simulink model "GolfSwing3D_SimscapePhysicalInterfaceSwitching"  (R2024b)
settings: Solver=VariableStepAuto  StartTime=0.0  StopTime=StopTime  MaxStep=0.001  RelTol=1e-3
model workspace: external: MAT-File 3DModelInputs.mat (data not in the file)
undefined symbols (not defined in the file): GripStrength, KillswitchFinalValue, KillswitchInitialValue, KillswitchStepTime, LeftLowerArmLength, PlaneTilt, RightLowerArmLength, UpperTorsoLength, X, Y, Z
libraries: nesl_utility x383, sm_lib x140, fl_lib x16, matrix_library x11, simulink x1
(part 9 of 14)

== system GolfSwing3D_SimscapePhysicalInterfaceSwitching/Right Scapula Joint/RScap Kinematically Driven ==
  Kinematically Driven RScap : sm_lib/Joints/Universal Joint  JointMode=Normal  CompositeWrenchDir=FollowerOnBase  CompositeWrenchFrame=BaseFrame  SenseConstraintForce=off  SenseConstraintTorque=off  SenseTotalForce=on  SenseTotalTorque=on  RxPositionTargetSpecify=off  RxPositionTargetPriority=Low  RxPositionTargetValue=RScapStartPositionX  RxPositionTargetValueUnits=deg  RxVelocityTargetSpecify=off  RxVelocityTargetPriority=Low  RxVelocityTargetValue=RScapStartVelocityX  RxVelocityTargetValueUnits=deg/s  RxEquilibriumPosition=0  RxEquilibriumPositionUnits=deg  RxSpringStiffness=0  RxSpringStiffnessUnits=N*m/deg  RxDampingCoefficient=0  RxDampingCoefficientUnits=N*m/(deg/s)  RxLowerLimitSpecify=off  RxLowerLimitBound=-30  RxLowerLimitBoundUnits=deg  RxLowerLimitStiffness=200  RxLowerLimitStiffnessUnits=N*m/deg  RxLowerLimitDamping=10  RxLowerLimitDampingUnits=N*m/(deg/s)  RxLowerLimitTransitionRegionWidth=0.1  RxLowerLimitTransitionRegionWidthUnits=deg  RxUpperLimitSpecify=off  RxUpperLimitBound=30  RxUpperLimitBoundUnits=deg  RxUpperLimitStiffness=200  RxUpperLimitStiffnessUnits=N*m/deg  RxUpperLimitDamping=10  RxUpperLimitDampingUnits=N*m/(deg/s)  RxUpperLimitTransitionRegionWidth=0.1  RxUpperLimitTransitionRegionWidthUnits=deg  RxTorqueActuationMode=ComputedTorque  RxMotionActuationMode=InputMotion  RxSensePosition=on  RxSenseVelocity=on  RxSenseAcceleration=off  RxSenseTorqueForce=on  RxSenseLowerLimitTorqueForce=off  RxSenseUpperLimitTorqueForce=off  RyPositionTargetSpecify=off  RyPositionTargetPriority=Low  RyPositionTargetValue=RScapStartPositionY  RyPositionTargetValueUnits=deg  RyVelocityTargetSpecify=off  RyVelocityTargetPriority=Low  RyVelocityTargetValue=RScapStartVelocityY  RyVelocityTargetValueUnits=deg/s  RyEquilibriumPosition=0  RyEquilibriumPositionUnits=deg  RySpringStiffness=0  RySpringStiffnessUnits=N*m/deg  RyDampingCoefficient=0  RyDampingCoefficientUnits=N*m/(deg/s)  RyLowerLimitSpecify=off  RyLowerLimitBound=-30  RyLowerLimitBoundUnits=deg  RyLowerLimitStiffness=200  RyLowerLimitStiffnessUnits=N*m/deg  RyLowerLimitDamping=10  RyLowerLimitDampingUnits=N*m/(deg/s)  RyLowerLimitTransitionRegionWidth=0.1  RyLowerLimitTransitionRegionWidthUnits=deg  RyUpperLimitSpecify=off  RyUpperLimitBound=30  RyUpperLimitBoundUnits=deg  RyUpperLimitStiffness=200  RyUpperLimitStiffnessUnits=N*m/deg  RyUpperLimitDamping=10  RyUpperLimitDampingUnits=N*m/(deg/s)  RyUpperLimitTransitionRegionWidth=0.1  RyUpperLimitTransitionRegionWidthUnits=deg  RyTorqueActuationMode=ComputedTorque  RyMotionActuationMode=InputMotion  RySensePosition=on  RySenseVelocity=on  RySenseAcceleration=off  RySenseTorqueForce=on  RySenseLowerLimitTorqueForce=off  RySenseUpperLimitTorqueForce=off
  RScapForceLocal : nesl_utility/PS-Simulink Converter  PhysicalDomain=network_engine_domain  SubClassName=ps_output  LeftPortType=input  RightPortType=output  PseudoPeriodic=off  Frequencies=[]  VectorFormat=1-D array  Unit=inherit  AffineConversion=off
  RScapPositionX : nesl_utility/PS-Simulink Converter  PhysicalDomain=network_engine_domain  SubClassName=ps_output  LeftPortType=input  RightPortType=output  PseudoPeriodic=off  Frequencies=[]  VectorFormat=1-D array  Unit=deg  AffineConversion=off
  RScapPositionY : nesl_utility/PS-Simulink Converter  PhysicalDomain=network_engine_domain  SubClassName=ps_output  LeftPortType=input  RightPortType=output  PseudoPeriodic=off  Frequencies=[]  VectorFormat=1-D array  Unit=deg  AffineConversion=off
  RScapTorqueLocal : nesl_utility/PS-Simulink Converter  PhysicalDomain=network_engine_domain  SubClassName=ps_output  LeftPortType=input  RightPortType=output  PseudoPeriodic=off  Frequencies=[]  VectorFormat=1-D array  Unit=inherit  AffineConversion=off
  RScapTorqueXInput : nesl_utility/PS-Simulink Converter  PhysicalDomain=network_engine_domain  SubClassName=ps_output  LeftPortType=input  RightPortType=output  PseudoPeriodic=off  Frequencies=[]  VectorFormat=1-D array  Unit=inherit  AffineConversion=off
  RScapTorqueYInput : nesl_utility/PS-Simulink Converter  PhysicalDomain=network_engine_domain  SubClassName=ps_output  LeftPortType=input  RightPortType=output  PseudoPeriodic=off  Frequencies=[]  VectorFormat=1-D array  Unit=inherit  AffineConversion=off
  RScapVelocityX : nesl_utility/PS-Simulink Converter  PhysicalDomain=network_engine_domain  SubClassName=ps_output  LeftPortType=input  RightPortType=output  PseudoPeriodic=off  Frequencies=[]  VectorFormat=1-D array  Unit=deg/s  AffineConversion=off
  RScapVelocityY : nesl_utility/PS-Simulink Converter  PhysicalDomain=network_engine_domain  SubClassName=ps_output  LeftPortType=input  RightPortType=output  PseudoPeriodic=off  Frequencies=[]  VectorFormat=1-D array  Unit=deg/s  AffineConversion=off
  Simulink-PS Converter14 : nesl_utility/Simulink-PS Converter  PhysicalDomain=network_engine_domain  SubClassName=ps_input  LeftPortType=input  RightPortType=output  PseudoPeriodic=off  Frequencies=[]  NoiseDistribution=none  NoiseParameters=[]  Unit=deg  AffineConversion=off  FilteringAndDerivatives=provide  SimscapeFilterOrder=1  InputFilterTimeConstant=0.001  UdotUserProvided=2
  Simulink-PS Converter15 : nesl_utility/Simulink-PS Converter  PhysicalDomain=network_engine_domain  SubClassName=ps_input  LeftPortType=input  RightPortType=output  PseudoPeriodic=off  Frequencies=[]  NoiseDistribution=none  NoiseParameters=[]  Unit=deg  AffineConversion=off  FilteringAndDerivatives=provide  SimscapeFilterOrder=1  InputFilterTimeConstant=0.001  UdotUserProvided=2
  Conn1 : PMIOPort  Side=Right
  Conn2 : PMIOPort  Port=2  Side=Left
  tag scope: RScapPositionX=global, RScapPositionY=global, RScapVelocityX=global, RScapVelocityY=global
  wires:
  [FcnOutRScapAccelerationY] -> Simulink-PS Converter15/3
  RScapPositionX/1 -> [RScapPositionX]  "RScapPositionX"
  RScapVelocityX/1 -> [RScapVelocityX]  "RScapVelocityX"
  [FcnOutRScapAccelerationX] -> Simulink-PS Converter14/3
  [FcnOutRScapPositionY] -> Simulink-PS Converter15/1
  RScapVelocityY/1 -> [RScapVelocityY]  "RScapVelocityY"
  RScapPositionY/1 -> [RScapPositionY]  "RScapPositionY"
  [FcnOutRScapPositionX] -> Simulink-PS Converter14/1
  [FcnOutRScapVelocityY] -> Simulink-PS Converter15/2
  [FcnOutRScapVelocityX] -> Simulink-PS Converter14/2
  RScapForceLocal/1 -> ?  "RScapForceLocal"
  RScapTorqueLocal/1 -> ?  "RScapTorqueLocal"
  RScapTorqueXInput/1 -> ?  "RScapTorqueXInput"
  RScapTorqueYInput/1 -> ?  "RScapTorqueYInput"
  connections:
  RScapVelocityX/LConn1 -- Kinematically Driven RScap/RConn3
  RScapPositionX/LConn1 -- Kinematically Driven RScap/RConn2
  Kinematically Driven RScap/RConn1 -- Conn1/RConn1
  RScapForceLocal/LConn1 -- Kinematically Driven RScap/RConn8
  Simulink-PS Converter15/RConn1 -- Kinematically Driven RScap/LConn3
  RScapVelocityY/LConn1 -- Kinematically Driven RScap/RConn6
  Simulink-PS Converter14/RConn1 -- Kinematically Driven RScap/LConn2
  RScapTorqueLocal/LConn1 -- Kinematically Driven RScap/RConn9
  RScapPositionY/LConn1 -- Kinematically Driven RScap/RConn5
  Kinematically Driven RScap/LConn1 -- Conn2/RConn1
  RScapTorqueYInput/LConn1 -- Kinematically Driven RScap/RConn7
  RScapTorqueXInput/LConn1 -- Kinematically Driven RScap/RConn4

== system GolfSwing3D_SimscapePhysicalInterfaceSwitching/Right Scapula Joint/RScap Kinetically Driven ==
  Kinetically Driven RScap : sm_lib/Joints/Universal Joint  JointMode=Normal  CompositeWrenchDir=FollowerOnBase  CompositeWrenchFrame=BaseFrame  SenseConstraintForce=off  SenseConstraintTorque=off  SenseTotalForce=on  SenseTotalTorque=on  RxPositionTargetSpecify=on  RxPositionTargetPriority=Low  RxPositionTargetValue=RScapStartPositionX  RxPositionTargetValueUnits=deg  RxVelocityTargetSpecify=off  RxVelocityTargetPriority=Low  RxVelocityTargetValue=RScapStartVelocityX  RxVelocityTargetValueUnits=deg/s  RxEquilibriumPosition=0  RxEquilibriumPositionUnits=deg  RxSpringStiffness=0  RxSpringStiffnessUnits=N*m/deg  RxDampingCoefficient=0  RxDampingCoefficientUnits=N*m/(deg/s)  RxLowerLimitSpecify=off  RxLowerLimitBound=-30  RxLowerLimitBoundUnits=deg  RxLowerLimitStiffness=200  RxLowerLimitStiffnessUnits=N*m/deg  RxLowerLimitDamping=10  RxLowerLimitDampingUnits=N*m/(deg/s)  RxLowerLimitTransitionRegionWidth=0.1  RxLowerLimitTransitionRegionWidthUnits=deg  RxUpperLimitSpecify=off  RxUpperLimitBound=30  RxUpperLimitBoundUnits=deg  RxUpperLimitStiffness=200  RxUpperLimitStiffnessUnits=N*m/deg  RxUpperLimitDamping=10  RxUpperLimitDampingUnits=N*m/(deg/s)  RxUpperLimitTransitionRegionWidth=0.1  RxUpperLimitTransitionRegionWidthUnits=deg  RxTorqueActuationMode=InputTorque  RxMotionActuationMode=ComputedMotion  RxSensePosition=on  RxSenseVelocity=on  RxSenseAcceleration=off  RxSenseTorqueForce=on  RxSenseLowerLimitTorqueForce=off  RxSenseUpperLimitTorqueForce=off  RyPositionTargetSpecify=on  RyPositionTargetPriority=Low  RyPositionTargetValue=RScapStartPositionY  RyPositionTargetValueUnits=deg  RyVelocityTargetSpecify=off  RyVelocityTargetPriority=Low  RyVelocityTargetValue=RScapStartVelocityY  RyVelocityTargetValueUnits=deg/s  RyEquilibriumPosition=0  RyEquilibriumPositionUnits=deg  RySpringStiffness=0  RySpringStiffnessUnits=N*m/deg  RyDampingCoefficient=0  RyDampingCoefficientUnits=N*m/(deg/s)  RyLowerLimitSpecify=off  RyLowerLimitBound=-30  RyLowerLimitBoundUnits=deg  RyLowerLimitStiffness=200  RyLowerLimitStiffnessUnits=N*m/deg  RyLowerLimitDamping=10  RyLowerLimitDampingUnits=N*m/(deg/s)  RyLowerLimitTransitionRegionWidth=0.1  RyLowerLimitTransitionRegionWidthUnits=deg  RyUpperLimitSpecify=off  RyUpperLimitBound=30  RyUpperLimitBoundUnits=deg  RyUpperLimitStiffness=200  RyUpperLimitStiffnessUnits=N*m/deg  RyUpperLimitDamping=10  RyUpperLimitDampingUnits=N*m/(deg/s)  RyUpperLimitTransitionRegionWidth=0.1  RyUpperLimitTransitionRegionWidthUnits=deg  RyTorqueActuationMode=InputTorque  RyMotionActuationMode=ComputedMotion  RySensePosition=on  RySenseVelocity=on  RySenseAcceleration=off  RySenseTorqueForce=on  RySenseLowerLimitTorqueForce=off  RySenseUpperLimitTorqueForce=off
  RScapForceLocal : nesl_utility/PS-Simulink Converter  PhysicalDomain=network_engine_domain  SubClassName=ps_output  LeftPortType=input  RightPortType=output  PseudoPeriodic=off  Frequencies=[]  VectorFormat=1-D array  Unit=inherit  AffineConversion=off
  RScapPositionX : nesl_utility/PS-Simulink Converter  PhysicalDomain=network_engine_domain  SubClassName=ps_output  LeftPortType=input  RightPortType=output  PseudoPeriodic=off  Frequencies=[]  VectorFormat=1-D array  Unit=deg  AffineConversion=off
  RScapPositionY : nesl_utility/PS-Simulink Converter  PhysicalDomain=network_engine_domain  SubClassName=ps_output  LeftPortType=input  RightPortType=output  PseudoPeriodic=off  Frequencies=[]  VectorFormat=1-D array  Unit=deg  AffineConversion=off
  RScapTorque : nesl_utility/PS-Simulink Converter  PhysicalDomain=network_engine_domain  SubClassName=ps_output  LeftPortType=input  RightPortType=output  PseudoPeriodic=off  Frequencies=[]  VectorFormat=1-D array  Unit=inherit  AffineConversion=off
  RScapTorqueXInput : nesl_utility/PS-Simulink Converter  PhysicalDomain=network_engine_domain  SubClassName=ps_output  LeftPortType=input  RightPortType=output  PseudoPeriodic=off  Frequencies=[]  VectorFormat=1-D array  Unit=inherit  AffineConversion=off
  RScapTorqueYInput : nesl_utility/PS-Simulink Converter  PhysicalDomain=network_engine_domain  SubClassName=ps_output  LeftPortType=input  RightPortType=output  PseudoPeriodic=off  Frequencies=[]  VectorFormat=1-D array  Unit=inherit  AffineConversion=off
  RScapVelocityX : nesl_utility/PS-Simulink Converter  PhysicalDomain=network_engine_domain  SubClassName=ps_output  LeftPortType=input  RightPortType=output  PseudoPeriodic=off  Frequencies=[]  VectorFormat=1-D array  Unit=deg/s  AffineConversion=off
  RScapVelocityY : nesl_utility/PS-Simulink Converter  PhysicalDomain=network_engine_domain  SubClassName=ps_output  LeftPortType=input  RightPortType=output  PseudoPeriodic=off  Frequencies=[]  VectorFormat=1-D array  Unit=deg/s  AffineConversion=off
  RightScapTorqueX : nesl_utility/Simulink-PS Converter  PhysicalDomain=network_engine_domain  SubClassName=ps_input  LeftPortType=input  RightPortType=output  PseudoPeriodic=off  Frequencies=[]  NoiseDistribution=none  NoiseParameters=[]  Unit=N*m  AffineConversion=off  FilteringAndDerivatives=provide  SimscapeFilterOrder=1  InputFilterTimeConstant=0.001  UdotUserProvided=0
  RightScapTorqueY : nesl_utility/Simulink-PS Converter  PhysicalDomain=network_engine_domain  SubClassName=ps_input  LeftPortType=input  RightPortType=output  PseudoPeriodic=off  Frequencies=[]  NoiseDistribution=none  NoiseParameters=[]  Unit=N*m  AffineConversion=off  FilteringAndDerivatives=provide  SimscapeFilterOrder=1  InputFilterTimeConstant=0.001  UdotUserProvided=0
  Conn1 : PMIOPort  Side=Left
  Conn2 : PMIOPort  Port=2  Side=Right
  tag scope: RScapPositionX=global, RScapPositionY=global, RScapVelocityX=global, RScapVelocityY=global
  wires:
  RScapPositionY/1 -> [RScapPositionY]  "RScapPositionY"
  [FcnOutRScapTorqueY] -> RightScapTorqueY/1
  [FcnOutRScapTorqueX] -> RightScapTorqueX/1
  RScapVelocityY/1 -> [RScapVelocityY]  "RScapVelocityY"
  RScapVelocityX/1 -> [RScapVelocityX]  "RScapVelocityX"
  RScapPositionX/1 -> [RScapPositionX]  "RScapPositionX"
  RScapTorque/1 -> ?  "RScapTorqueLocal"
  RScapForceLocal/1 -> ?  "RScapForceLocal"
  RScapTorqueXInput/1 -> ?  "RScapTorqueXInput"
  RScapTorqueYInput/1 -> ?  "RScapTorqueYInput"
  connections:
  Kinetically Driven RScap/LConn2 -- RightScapTorqueX/RConn1
  Kinetically Driven RScap/RConn3 -- RScapVelocityX/LConn1
  Kinetically Driven RScap/RConn6 -- RScapVelocityY/LConn1
  RScapForceLocal/LConn1 -- Kinetically Driven RScap/RConn8
  RScapTorque/LConn1 -- Kinetically Driven RScap/RConn9
  Kinetically Driven RScap/RConn2 -- RScapPositionX/LConn1
  RightScapTorqueY/RConn1 -- Kinetically Driven RScap/LConn3
  Kinetically Driven RScap/RConn5 -- RScapPositionY/LConn1
  Kinetically Driven RScap/LConn1 -- Conn1/RConn1
  Conn2/RConn1 -- Kinetically Driven RScap/RConn1
  RScapTorqueXInput/LConn1 -- Kinetically Driven RScap/RConn4
  RScapTorqueYInput/LConn1 -- Kinetically Driven RScap/RConn7

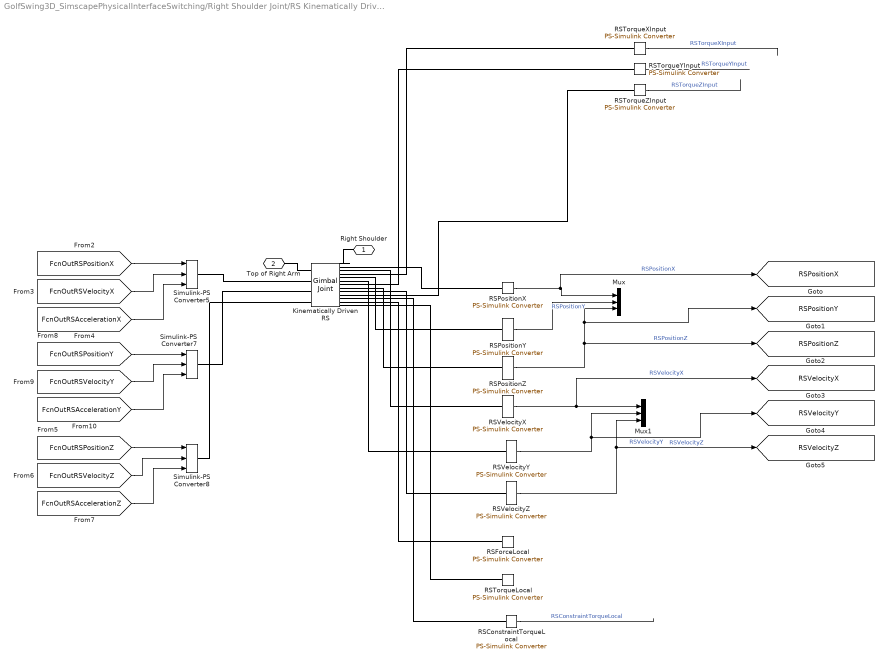
== system GolfSwing3D_SimscapePhysicalInterfaceSwitching/Right Shoulder Joint/RS Kinematically Driven ==
  Kinematically Driven RS : sm_lib/Joints/Gimbal Joint  JointMode=Normal  CompositeWrenchDir=BaseOnFollower  CompositeWrenchFrame=FollowerFrame  SenseConstraintForce=off  SenseConstraintTorque=on  SenseTotalForce=on  SenseTotalTorque=on  RxPositionTargetSpecify=off  RxPositionTargetPriority=Low  RxPositionTargetValue=RSStartPositionX  RxPositionTargetValueUnits=deg  RxVelocityTargetSpecify=off  RxVelocityTargetPriority=Low  RxVelocityTargetValue=RSStartVelocityX  RxVelocityTargetValueUnits=deg/s  RxEquilibriumPosition=120  RxEquilibriumPositionUnits=deg  RxSpringStiffness=0  RxSpringStiffnessUnits=N*m/deg  RxDampingCoefficient=0  RxDampingCoefficientUnits=N*m/(deg/s)  RxLowerLimitSpecify=off  RxLowerLimitBound=-45  RxLowerLimitBoundUnits=deg  RxLowerLimitStiffness=100  RxLowerLimitStiffnessUnits=N*m/deg  RxLowerLimitDamping=10  RxLowerLimitDampingUnits=N*m/(deg/s)  RxLowerLimitTransitionRegionWidth=0.1  RxLowerLimitTransitionRegionWidthUnits=deg  RxUpperLimitSpecify=off  RxUpperLimitBound=45  RxUpperLimitBoundUnits=deg  RxUpperLimitStiffness=100  RxUpperLimitStiffnessUnits=N*m/deg  RxUpperLimitDamping=10  RxUpperLimitDampingUnits=N*m/(deg/s)  RxUpperLimitTransitionRegionWidth=0.1  RxUpperLimitTransitionRegionWidthUnits=deg  RxTorqueActuationMode=ComputedTorque  RxMotionActuationMode=InputMotion  RxSensePosition=on  RxSenseVelocity=on  RxSenseAcceleration=off  RxSenseTorqueForce=on  RxSenseLowerLimitTorqueForce=off  RxSenseUpperLimitTorqueForce=off  RyPositionTargetSpecify=off  RyPositionTargetPriority=Low  RyPositionTargetValue=RSStartPositionY  RyPositionTargetValueUnits=deg  RyVelocityTargetSpecify=off  RyVelocityTargetPriority=Low  RyVelocityTargetValue=RSStartVelocityY  RyVelocityTargetValueUnits=deg/s  RyEquilibriumPosition=0  RyEquilibriumPositionUnits=deg  RySpringStiffness=0  RySpringStiffnessUnits=N*m/deg  RyDampingCoefficient=0  RyDampingCoefficientUnits=N*m/(deg/s)  RyLowerLimitSpecify=off  RyLowerLimitBound=-80  RyLowerLimitBoundUnits=deg  RyLowerLimitStiffness=100  RyLowerLimitStiffnessUnits=N*m/deg  RyLowerLimitDamping=10  RyLowerLimitDampingUnits=N*m/(deg/s)  RyLowerLimitTransitionRegionWidth=0.1  RyLowerLimitTransitionRegionWidthUnits=deg  RyUpperLimitSpecify=off  RyUpperLimitBound=80  RyUpperLimitBoundUnits=deg  RyUpperLimitStiffness=100  RyUpperLimitStiffnessUnits=N*m/deg  RyUpperLimitDamping=10  RyUpperLimitDampingUnits=N*m/(deg/s)  RyUpperLimitTransitionRegionWidth=0.1  RyUpperLimitTransitionRegionWidthUnits=deg  RyTorqueActuationMode=ComputedTorque  RyMotionActuationMode=InputMotion  RySensePosition=on  RySenseVelocity=on  RySenseAcceleration=off  RySenseTorqueForce=on  RySenseLowerLimitTorqueForce=off  RySenseUpperLimitTorqueForce=off  RzPositionTargetSpecify=off  RzPositionTargetPriority=Low  RzPositionTargetValue=RSStartPositionZ  RzPositionTargetValueUnits=deg  RzVelocityTargetSpecify=off  RzVelocityTargetPriority=Low  RzVelocityTargetValue=RSStartVelocityZ  RzVelocityTargetValueUnits=deg/s  RzEquilibriumPosition=0  RzEquilibriumPositionUnits=deg  RzSpringStiffness=0  RzSpringStiffnessUnits=N*m/deg  RzDampingCoefficient=0  RzDampingCoefficientUnits=N*m/(deg/s)  RzLowerLimitSpecify=off  RzLowerLimitBound=-120  RzLowerLimitBoundUnits=deg  RzLowerLimitStiffness=100  RzLowerLimitStiffnessUnits=N*m/deg  RzLowerLimitDamping=10  RzLowerLimitDampingUnits=N*m/(deg/s)  RzLowerLimitTransitionRegionWidth=0.1  RzLowerLimitTransitionRegionWidthUnits=deg  RzUpperLimitSpecify=off  RzUpperLimitBound=0  RzUpperLimitBoundUnits=deg  RzUpperLimitStiffness=100  RzUpperLimitStiffnessUnits=N*m/deg  RzUpperLimitDamping=10  RzUpperLimitDampingUnits=N*m/(deg/s)  RzUpperLimitTransitionRegionWidth=0.1  RzUpperLimitTransitionRegionWidthUnits=deg  RzTorqueActuationMode=ComputedTorque  RzMotionActuationMode=InputMotion  RzSensePosition=on  RzSenseVelocity=on  RzSenseAcceleration=off  RzSenseTorqueForce=on  RzSenseLowerLimitTorqueForce=off  RzSenseUpperLimitTorqueForce=off
  Mux : Mux  Inputs=3
  Mux1 : Mux  Inputs=3
  RSConstraintTorqueLocal : nesl_utility/PS-Simulink Converter  PhysicalDomain=network_engine_domain  SubClassName=ps_output  LeftPortType=input  RightPortType=output  PseudoPeriodic=off  Frequencies=[]  VectorFormat=1-D array  Unit=inherit  AffineConversion=off
  RSForceLocal : nesl_utility/PS-Simulink Converter  PhysicalDomain=network_engine_domain  SubClassName=ps_output  LeftPortType=input  RightPortType=output  PseudoPeriodic=off  Frequencies=[]  VectorFormat=1-D array  Unit=inherit  AffineConversion=off
  RSPositionX : nesl_utility/PS-Simulink Converter  PhysicalDomain=network_engine_domain  SubClassName=ps_output  LeftPortType=input  RightPortType=output  PseudoPeriodic=off  Frequencies=[]  VectorFormat=1-D array  Unit=deg  AffineConversion=off
  RSPositionY : nesl_utility/PS-Simulink Converter  PhysicalDomain=network_engine_domain  SubClassName=ps_output  LeftPortType=input  RightPortType=output  PseudoPeriodic=off  Frequencies=[]  VectorFormat=1-D array  Unit=deg  AffineConversion=off
  RSPositionZ : nesl_utility/PS-Simulink Converter  PhysicalDomain=network_engine_domain  SubClassName=ps_output  LeftPortType=input  RightPortType=output  PseudoPeriodic=off  Frequencies=[]  VectorFormat=1-D array  Unit=deg  AffineConversion=off
  RSTorqueLocal : nesl_utility/PS-Simulink Converter  PhysicalDomain=network_engine_domain  SubClassName=ps_output  LeftPortType=input  RightPortType=output  PseudoPeriodic=off  Frequencies=[]  VectorFormat=1-D array  Unit=inherit  AffineConversion=off
  RSTorqueXInput : nesl_utility/PS-Simulink Converter  PhysicalDomain=network_engine_domain  SubClassName=ps_output  LeftPortType=input  RightPortType=output  PseudoPeriodic=off  Frequencies=[]  VectorFormat=1-D array  Unit=inherit  AffineConversion=off
  RSTorqueYInput : nesl_utility/PS-Simulink Converter  PhysicalDomain=network_engine_domain  SubClassName=ps_output  LeftPortType=input  RightPortType=output  PseudoPeriodic=off  Frequencies=[]  VectorFormat=1-D array  Unit=inherit  AffineConversion=off
  RSTorqueZInput : nesl_utility/PS-Simulink Converter  PhysicalDomain=network_engine_domain  SubClassName=ps_output  LeftPortType=input  RightPortType=output  PseudoPeriodic=off  Frequencies=[]  VectorFormat=1-D array  Unit=inherit  AffineConversion=off
  RSVelocityX : nesl_utility/PS-Simulink Converter  PhysicalDomain=network_engine_domain  SubClassName=ps_output  LeftPortType=input  RightPortType=output  PseudoPeriodic=off  Frequencies=[]  VectorFormat=1-D array  Unit=deg/s  AffineConversion=off
  RSVelocityY : nesl_utility/PS-Simulink Converter  PhysicalDomain=network_engine_domain  SubClassName=ps_output  LeftPortType=input  RightPortType=output  PseudoPeriodic=off  Frequencies=[]  VectorFormat=1-D array  Unit=deg/s  AffineConversion=off
  RSVelocityZ : nesl_utility/PS-Simulink Converter  PhysicalDomain=network_engine_domain  SubClassName=ps_output  LeftPortType=input  RightPortType=output  PseudoPeriodic=off  Frequencies=[]  VectorFormat=1-D array  Unit=deg/s  AffineConversion=off
  Simulink-PS Converter5 : nesl_utility/Simulink-PS Converter  PhysicalDomain=network_engine_domain  SubClassName=ps_input  LeftPortType=input  RightPortType=output  PseudoPeriodic=off  Frequencies=[]  NoiseDistribution=none  NoiseParameters=[]  Unit=deg  AffineConversion=off  FilteringAndDerivatives=provide  SimscapeFilterOrder=1  InputFilterTimeConstant=0.001  UdotUserProvided=2
  Simulink-PS Converter7 : nesl_utility/Simulink-PS Converter  PhysicalDomain=network_engine_domain  SubClassName=ps_input  LeftPortType=input  RightPortType=output  PseudoPeriodic=off  Frequencies=[]  NoiseDistribution=none  NoiseParameters=[]  Unit=deg  AffineConversion=off  FilteringAndDerivatives=provide  SimscapeFilterOrder=1  InputFilterTimeConstant=0.001  UdotUserProvided=2
  Simulink-PS Converter8 : nesl_utility/Simulink-PS Converter  PhysicalDomain=network_engine_domain  SubClassName=ps_input  LeftPortType=input  RightPortType=output  PseudoPeriodic=off  Frequencies=[]  NoiseDistribution=none  NoiseParameters=[]  Unit=deg  AffineConversion=off  FilteringAndDerivatives=provide  SimscapeFilterOrder=1  InputFilterTimeConstant=0.001  UdotUserProvided=2
  Right Shoulder : PMIOPort  Side=Right
  Top of Right Arm : PMIOPort  Port=2  Side=Left
  tag scope: RSPositionX=global, RSPositionY=global, RSPositionZ=global, RSVelocityX=global, RSVelocityY=global, RSVelocityZ=global
  wires:
  [FcnOutRSPositionY] -> Simulink-PS Converter7/1
  [FcnOutRSVelocityZ] -> Simulink-PS Converter8/2
  [FcnOutRSAccelerationZ] -> Simulink-PS Converter8/3
  [FcnOutRSAccelerationY] -> Simulink-PS Converter7/3
  [FcnOutRSPositionZ] -> Simulink-PS Converter8/1
  [FcnOutRSPositionX] -> Simulink-PS Converter5/1
  [FcnOutRSVelocityX] -> Simulink-PS Converter5/2
  [FcnOutRSAccelerationX] -> Simulink-PS Converter5/3
  [FcnOutRSVelocityY] -> Simulink-PS Converter7/2
  RSVelocityZ/1 -> [RSVelocityZ], Mux1/3  "RSVelocityZ"
  RSPositionZ/1 -> [RSPositionZ], [RSPositionY], Mux/3  "RSPositionZ"
  RSVelocityX/1 -> [RSVelocityX], Mux1/1  "RSVelocityX"
  RSVelocityY/1 -> Mux1/2, [RSVelocityY]  "RSVelocityY"
  RSPositionY/1 -> Mux/2  "RSPositionY"
  RSPositionX/1 -> [RSPositionX], Mux/1  "RSPositionX"
  RSConstraintTorqueLocal/1 -> ?  "RSConstraintTorqueLocal"
  RSTorqueYInput/1 -> ?  "RSTorqueYInput"
  RSTorqueXInput/1 -> ?  "RSTorqueXInput"
  RSTorqueZInput/1 -> ?  "RSTorqueZInput"
  connections:
  Simulink-PS Converter5/RConn1 -- Kinematically Driven RS/LConn2
  Simulink-PS Converter7/RConn1 -- Kinematically Driven RS/LConn3
  Simulink-PS Converter8/RConn1 -- Kinematically Driven RS/LConn4
  Kinematically Driven RS/RConn1 -- Right Shoulder/RConn1
  Kinematically Driven RS/LConn1 -- Top of Right Arm/RConn1
  Kinematically Driven RS/RConn2 -- RSPositionX/LConn1
  Kinematically Driven RS/RConn3 -- RSVelocityX/LConn1
  Kinematically Driven RS/RConn5 -- RSPositionY/LConn1
  Kinematically Driven RS/RConn6 -- RSVelocityY/LConn1
  Kinematically Driven RS/RConn8 -- RSPositionZ/LConn1
  Kinematically Driven RS/RConn9 -- RSVelocityZ/LConn1
  RSForceLocal/LConn1 -- Kinematically Driven RS/RConn12
  RSTorqueLocal/LConn1 -- Kinematically Driven RS/RConn13
  Kinematically Driven RS/RConn11 -- RSConstraintTorqueLocal/LConn1
  RSTorqueZInput/LConn1 -- Kinematically Driven RS/RConn10
  RSTorqueXInput/LConn1 -- Kinematically Driven RS/RConn4
  RSTorqueYInput/LConn1 -- Kinematically Driven RS/RConn7

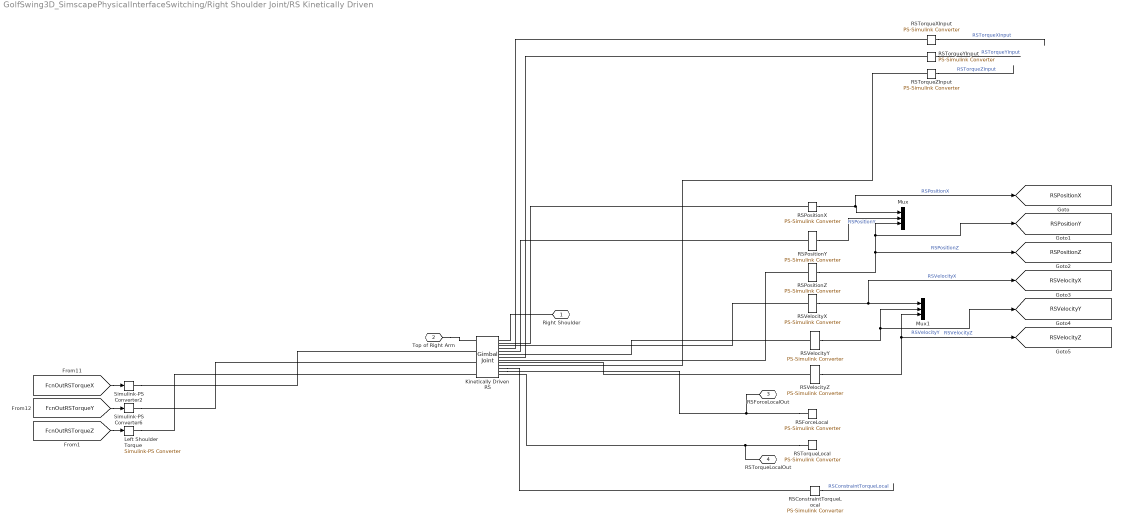
== system GolfSwing3D_SimscapePhysicalInterfaceSwitching/Right Shoulder Joint/RS Kinetically Driven ==
  Kinetically Driven RS : sm_lib/Joints/Gimbal Joint  JointMode=Normal  CompositeWrenchDir=BaseOnFollower  CompositeWrenchFrame=FollowerFrame  SenseConstraintForce=off  SenseConstraintTorque=on  SenseTotalForce=on  SenseTotalTorque=on  RxPositionTargetSpecify=on  RxPositionTargetPriority=Low  RxPositionTargetValue=RSStartPositionX  RxPositionTargetValueUnits=deg  RxVelocityTargetSpecify=off  RxVelocityTargetPriority=Low  RxVelocityTargetValue=RSStartVelocityX  RxVelocityTargetValueUnits=deg/s  RxEquilibriumPosition=120  RxEquilibriumPositionUnits=deg  RxSpringStiffness=0  RxSpringStiffnessUnits=N*m/deg  RxDampingCoefficient=0  RxDampingCoefficientUnits=N*m/(deg/s)  RxLowerLimitSpecify=off  RxLowerLimitBound=-45  RxLowerLimitBoundUnits=deg  RxLowerLimitStiffness=100  RxLowerLimitStiffnessUnits=N*m/deg  RxLowerLimitDamping=10  RxLowerLimitDampingUnits=N*m/(deg/s)  RxLowerLimitTransitionRegionWidth=0.1  RxLowerLimitTransitionRegionWidthUnits=deg  RxUpperLimitSpecify=off  RxUpperLimitBound=45  RxUpperLimitBoundUnits=deg  RxUpperLimitStiffness=100  RxUpperLimitStiffnessUnits=N*m/deg  RxUpperLimitDamping=10  RxUpperLimitDampingUnits=N*m/(deg/s)  RxUpperLimitTransitionRegionWidth=0.1  RxUpperLimitTransitionRegionWidthUnits=deg  RxTorqueActuationMode=InputTorque  RxMotionActuationMode=ComputedMotion  RxSensePosition=on  RxSenseVelocity=on  RxSenseAcceleration=off  RxSenseTorqueForce=on  RxSenseLowerLimitTorqueForce=off  RxSenseUpperLimitTorqueForce=off  RyPositionTargetSpecify=on  RyPositionTargetPriority=Low  RyPositionTargetValue=RSStartPositionY  RyPositionTargetValueUnits=deg  RyVelocityTargetSpecify=off  RyVelocityTargetPriority=Low  RyVelocityTargetValue=RSStartVelocityY  RyVelocityTargetValueUnits=deg/s  RyEquilibriumPosition=0  RyEquilibriumPositionUnits=deg  RySpringStiffness=0  RySpringStiffnessUnits=N*m/deg  RyDampingCoefficient=0  RyDampingCoefficientUnits=N*m/(deg/s)  RyLowerLimitSpecify=off  RyLowerLimitBound=-80  RyLowerLimitBoundUnits=deg  RyLowerLimitStiffness=100  RyLowerLimitStiffnessUnits=N*m/deg  RyLowerLimitDamping=10  RyLowerLimitDampingUnits=N*m/(deg/s)  RyLowerLimitTransitionRegionWidth=0.1  RyLowerLimitTransitionRegionWidthUnits=deg  RyUpperLimitSpecify=off  RyUpperLimitBound=80  RyUpperLimitBoundUnits=deg  RyUpperLimitStiffness=100  RyUpperLimitStiffnessUnits=N*m/deg  RyUpperLimitDamping=10  RyUpperLimitDampingUnits=N*m/(deg/s)  RyUpperLimitTransitionRegionWidth=0.1  RyUpperLimitTransitionRegionWidthUnits=deg  RyTorqueActuationMode=InputTorque  RyMotionActuationMode=ComputedMotion  RySensePosition=on  RySenseVelocity=on  RySenseAcceleration=off  RySenseTorqueForce=on  RySenseLowerLimitTorqueForce=off  RySenseUpperLimitTorqueForce=off  RzPositionTargetSpecify=on  RzPositionTargetPriority=Low  RzPositionTargetValue=RSStartPositionZ  RzPositionTargetValueUnits=deg  RzVelocityTargetSpecify=off  RzVelocityTargetPriority=Low  RzVelocityTargetValue=RSStartVelocityZ  RzVelocityTargetValueUnits=deg/s  RzEquilibriumPosition=0  RzEquilibriumPositionUnits=deg  RzSpringStiffness=0  RzSpringStiffnessUnits=N*m/deg  RzDampingCoefficient=0  RzDampingCoefficientUnits=N*m/(deg/s)  RzLowerLimitSpecify=off  RzLowerLimitBound=-120  RzLowerLimitBoundUnits=deg  RzLowerLimitStiffness=100  RzLowerLimitStiffnessUnits=N*m/deg  RzLowerLimitDamping=10  RzLowerLimitDampingUnits=N*m/(deg/s)  RzLowerLimitTransitionRegionWidth=0.1  RzLowerLimitTransitionRegionWidthUnits=deg  RzUpperLimitSpecify=off  RzUpperLimitBound=0  RzUpperLimitBoundUnits=deg  RzUpperLimitStiffness=100  RzUpperLimitStiffnessUnits=N*m/deg  RzUpperLimitDamping=10  RzUpperLimitDampingUnits=N*m/(deg/s)  RzUpperLimitTransitionRegionWidth=0.1  RzUpperLimitTransitionRegionWidthUnits=deg  RzTorqueActuationMode=InputTorque  RzMotionActuationMode=ComputedMotion  RzSensePosition=on  RzSenseVelocity=on  RzSenseAcceleration=off  RzSenseTorqueForce=on  RzSenseLowerLimitTorqueForce=off  RzSenseUpperLimitTorqueForce=off
  Left Shoulder Torque : nesl_utility/Simulink-PS Converter  PhysicalDomain=network_engine_domain  SubClassName=ps_input  LeftPortType=input  RightPortType=output  PseudoPeriodic=off  Frequencies=[]  NoiseDistribution=none  NoiseParameters=[]  Unit=N*m  AffineConversion=off  FilteringAndDerivatives=provide  SimscapeFilterOrder=1  InputFilterTimeConstant=0.001  UdotUserProvided=0
  Mux : Mux  Inputs=3
  Mux1 : Mux  Inputs=3
  RSConstraintTorqueLocal : nesl_utility/PS-Simulink Converter  PhysicalDomain=network_engine_domain  SubClassName=ps_output  LeftPortType=input  RightPortType=output  PseudoPeriodic=off  Frequencies=[]  VectorFormat=1-D array  Unit=inherit  AffineConversion=off
  RSForceLocal : nesl_utility/PS-Simulink Converter  PhysicalDomain=network_engine_domain  SubClassName=ps_output  LeftPortType=input  RightPortType=output  PseudoPeriodic=off  Frequencies=[]  VectorFormat=1-D array  Unit=inherit  AffineConversion=off
  RSPositionX : nesl_utility/PS-Simulink Converter  PhysicalDomain=network_engine_domain  SubClassName=ps_output  LeftPortType=input  RightPortType=output  PseudoPeriodic=off  Frequencies=[]  VectorFormat=1-D array  Unit=deg  AffineConversion=off
  RSPositionY : nesl_utility/PS-Simulink Converter  PhysicalDomain=network_engine_domain  SubClassName=ps_output  LeftPortType=input  RightPortType=output  PseudoPeriodic=off  Frequencies=[]  VectorFormat=1-D array  Unit=deg  AffineConversion=off
  RSPositionZ : nesl_utility/PS-Simulink Converter  PhysicalDomain=network_engine_domain  SubClassName=ps_output  LeftPortType=input  RightPortType=output  PseudoPeriodic=off  Frequencies=[]  VectorFormat=1-D array  Unit=deg  AffineConversion=off
  RSTorqueLocal : nesl_utility/PS-Simulink Converter  PhysicalDomain=network_engine_domain  SubClassName=ps_output  LeftPortType=input  RightPortType=output  PseudoPeriodic=off  Frequencies=[]  VectorFormat=1-D array  Unit=inherit  AffineConversion=off
  RSTorqueXInput : nesl_utility/PS-Simulink Converter  PhysicalDomain=network_engine_domain  SubClassName=ps_output  LeftPortType=input  RightPortType=output  PseudoPeriodic=off  Frequencies=[]  VectorFormat=1-D array  Unit=inherit  AffineConversion=off
  RSTorqueYInput : nesl_utility/PS-Simulink Converter  PhysicalDomain=network_engine_domain  SubClassName=ps_output  LeftPortType=input  RightPortType=output  PseudoPeriodic=off  Frequencies=[]  VectorFormat=1-D array  Unit=inherit  AffineConversion=off
  RSTorqueZInput : nesl_utility/PS-Simulink Converter  PhysicalDomain=network_engine_domain  SubClassName=ps_output  LeftPortType=input  RightPortType=output  PseudoPeriodic=off  Frequencies=[]  VectorFormat=1-D array  Unit=inherit  AffineConversion=off
  RSVelocityX : nesl_utility/PS-Simulink Converter  PhysicalDomain=network_engine_domain  SubClassName=ps_output  LeftPortType=input  RightPortType=output  PseudoPeriodic=off  Frequencies=[]  VectorFormat=1-D array  Unit=deg/s  AffineConversion=off
  RSVelocityY : nesl_utility/PS-Simulink Converter  PhysicalDomain=network_engine_domain  SubClassName=ps_output  LeftPortType=input  RightPortType=output  PseudoPeriodic=off  Frequencies=[]  VectorFormat=1-D array  Unit=deg/s  AffineConversion=off
  RSVelocityZ : nesl_utility/PS-Simulink Converter  PhysicalDomain=network_engine_domain  SubClassName=ps_output  LeftPortType=input  RightPortType=output  PseudoPeriodic=off  Frequencies=[]  VectorFormat=1-D array  Unit=deg/s  AffineConversion=off
  Simulink-PS Converter2 : nesl_utility/Simulink-PS Converter  PhysicalDomain=network_engine_domain  SubClassName=ps_input  LeftPortType=input  RightPortType=output  PseudoPeriodic=off  Frequencies=[]  NoiseDistribution=none  NoiseParameters=[]  Unit=1  AffineConversion=off  FilteringAndDerivatives=provide  SimscapeFilterOrder=1  InputFilterTimeConstant=0.001  UdotUserProvided=0
  Simulink-PS Converter6 : nesl_utility/Simulink-PS Converter  PhysicalDomain=network_engine_domain  SubClassName=ps_input  LeftPortType=input  RightPortType=output  PseudoPeriodic=off  Frequencies=[]  NoiseDistribution=none  NoiseParameters=[]  Unit=1  AffineConversion=off  FilteringAndDerivatives=provide  SimscapeFilterOrder=1  InputFilterTimeConstant=0.001  UdotUserProvided=0
  Right Shoulder : PMIOPort  Side=Right
  Top of Right Arm : PMIOPort  Port=2  Side=Left
  RSForceLocalOut : PMIOPort  Port=3  Side=Right
  RSTorqueLocalOut : PMIOPort  Port=4  Side=Right
  tag scope: RSPositionX=global, RSPositionY=global, RSPositionZ=global, RSVelocityX=global, RSVelocityY=global, RSVelocityZ=global
  wires:
  [FcnOutRSTorqueZ] -> Left Shoulder Torque/1
  RSPositionX/1 -> [RSPositionX], Mux/1  "RSPositionX"
  [FcnOutRSTorqueY] -> Simulink-PS Converter6/1
  RSVelocityY/1 -> Mux1/2, [RSVelocityY]  "RSVelocityY"
  RSPositionY/1 -> Mux/2  "RSPositionY"
  RSVelocityZ/1 -> [RSVelocityZ], Mux1/3  "RSVelocityZ"
  [FcnOutRSTorqueX] -> Simulink-PS Converter2/1
  RSVelocityX/1 -> [RSVelocityX], Mux1/1  "RSVelocityX"
  RSPositionZ/1 -> [RSPositionZ], [RSPositionY], Mux/3  "RSPositionZ"
  RSConstraintTorqueLocal/1 -> ?  "RSConstraintTorqueLocal"
  RSTorqueXInput/1 -> ?  "RSTorqueXInput"
  RSTorqueZInput/1 -> ?  "RSTorqueZInput"
  RSTorqueYInput/1 -> ?  "RSTorqueYInput"
  connections:
  RSVelocityY/LConn1 -- Kinetically Driven RS/RConn6
  Left Shoulder Torque/RConn1 -- Kinetically Driven RS/LConn4
  RSTorqueLocal/LConn1 -- Kinetically Driven RS/RConn13 -- RSTorqueLocalOut/RConn1
  RSPositionY/LConn1 -- Kinetically Driven RS/RConn5
  RSPositionZ/LConn1 -- Kinetically Driven RS/RConn8
  Simulink-PS Converter2/RConn1 -- Kinetically Driven RS/LConn2
  RSVelocityX/LConn1 -- Kinetically Driven RS/RConn3
  Simulink-PS Converter6/RConn1 -- Kinetically Driven RS/LConn3
  RSPositionX/LConn1 -- Kinetically Driven RS/RConn2
  RSForceLocal/LConn1 -- Kinetically Driven RS/RConn12 -- RSForceLocalOut/RConn1
  RSVelocityZ/LConn1 -- Kinetically Driven RS/RConn9
  Top of Right Arm/RConn1 -- Kinetically Driven RS/LConn1
  Right Shoulder/RConn1 -- Kinetically Driven RS/RConn1
  Kinetically Driven RS/RConn11 -- RSConstraintTorqueLocal/LConn1
  RSTorqueYInput/LConn1 -- Kinetically Driven RS/RConn7
  RSTorqueZInput/LConn1 -- Kinetically Driven RS/RConn10
  RSTorqueXInput/LConn1 -- Kinetically Driven RS/RConn4

== system GolfSwing3D_SimscapePhysicalInterfaceSwitching/Right Upper Arm/Right Upper Arm MOF ==
  R Vector Elbow Force on Right Arm : Sum  Inputs=-+
  R Vector Shoulder Force on Right Arm : Sum  Inputs=-+
  RElbowonRArmMOFGlobal : matrix_library/Cross Product
  RElbowonRArmMOFLocal : Product  Multiplication=Matrix(*)
  RSAngularImpulseonArm : Integrator
  RShoulderonRArmMOFGlobal : matrix_library/Cross Product
  RShoulderonRArmMOFLocal : Product  Multiplication=Matrix(*)
  RUACOM : sm_lib/Body Elements/Inertia Sensor  SensorExtent=BodyGroup  SpanWeldJoints=off  ExcludeGroundedBodies=off  MeasurementFrame=World  SenseMass=off  SenseCenterOfMass=on  SenseInertiaMatrix=off  SenseCenteredInertiaMatrix=off  SensePrincipalInertiaMatrix=off  SenseRotationMatrix=off  GraphicType=None  PrincipalInertiaFrameSize=20  GraphicVisPropType=SimpleVisualProperties  GraphicDiffuseColor=[0.5 0.5 0.5]  GraphicOpacity=1  GraphicSpecularColor=[0.5 0.5 0.5 1.0]  GraphicAmbientColor=[0.15 0.15 0.15 1.0]  GraphicEmissiveColor=[0.0 0.0 0.0 1.0]  GraphicShininess=75
  Right Upper Arm COM : nesl_utility/PS-Simulink Converter  PhysicalDomain=network_engine_domain  SubClassName=ps_output  LeftPortType=input  RightPortType=output  PseudoPeriodic=off  Frequencies=[]  VectorFormat=1-D array  Unit=inherit  AffineConversion=off
  Rotation Transform Right Arm : nesl_utility/PS-Simulink Converter  PhysicalDomain=network_engine_domain  SubClassName=ps_output  LeftPortType=input  RightPortType=output  PseudoPeriodic=off  Frequencies=[]  VectorFormat=1-D array  Unit=inherit  AffineConversion=off
  SumofMomentsRArmLocal : Product  Multiplication=Matrix(*)
  SumofMomentsRSonRArm : Sum
  SumofMomentsRightArmGlobal : Sum  Inputs=++++
  Transform Sensor : sm_lib/Frames and Transforms/Transform Sensor  MeasurementFrame=World  RotationSequence=XYX  SenseAngle=off  SenseAxis=off  SenseQ=off  SenseR=on  SenseRotationSequence=off  SenseOmegaX=off  SenseOmegaY=off  SenseOmegaZ=off  SenseOmega=off  SenseQDot=off  SenseRDot=off  SenseRotationSequenceDot=off  SenseAlphaX=off  SenseAlphaY=off  SenseAlphaZ=off  SenseAlpha=off  SenseQDDot=off  SenseRDDot=off  SenseX=off  SenseY=off  SenseZ=off  SenseXYZ=off  SenseRad=off  SenseAzim=off  SenseDist=off  SenseInc=off  SenseXDot=off  SenseYDot=off  SenseZDot=off  SenseXYZDot=off  SenseRadDot=off  SenseAzimDot=off  SenseDistDot=off  SenseIncDot=off  SenseXDDot=off  SenseYDDot=off  SenseZDDot=off  SenseXYZDDot=off  SenseRadDDot=off  SenseAzimDDot=off  SenseDistDDot=off  SenseIncDDot=off
  World Frame : sm_lib/Frames and Transforms/World Frame
  RightUpper  Arm : PMIOPort  Side=Left
  wires:
  Right Upper Arm COM/1 -> R Vector Elbow Force on Right Arm/1, R Vector Shoulder Force on Right Arm/1  "RUpperArmCOM"
  [RSGlobalPosition] -> R Vector Shoulder Force on Right Arm/2
  [REGlobalPosition] -> R Vector Elbow Force on Right Arm/2
  [RSonRArmFGlobalOut] -> RShoulderonRArmMOFGlobal/2
  R Vector Elbow Force on Right Arm/1 -> RElbowonRArmMOFGlobal/1
  [RForearmonRArmTGlobalOut] -> SumofMomentsRightArmGlobal/4
  [RForearmonRArmFGlobalOut] -> RElbowonRArmMOFGlobal/2
  R Vector Shoulder Force on Right Arm/1 -> RShoulderonRArmMOFGlobal/1
  SumofMomentsRightArmGlobal/1 -> SumofMomentsRArmLocal/2  "SumofMomentsRightArmGlobal"
  RElbowonRArmMOFGlobal/1 -> RElbowonRArmMOFLocal/2, SumofMomentsRightArmGlobal/2  "RElbowonRArmMOFGlobal"
  Rotation Transform Right Arm/1 -> SumofMomentsRArmLocal/1, RElbowonRArmMOFLocal/1, RShoulderonRArmMOFLocal/1
  RShoulderonRArmMOFGlobal/1 -> SumofMomentsRightArmGlobal/1, SumofMomentsRSonRArm/2, RShoulderonRArmMOFLocal/2  "RShoulderonRArmMOFGlobal"
  SumofMomentsRSonRArm/1 -> RSAngularImpulseonArm/1  "SumofMomentsRSonRArm"
  [RSonRArmTGlobalOut] -> SumofMomentsRSonRArm/1, SumofMomentsRightArmGlobal/3
  connections:
  RUACOM/LConn1 -- Transform Sensor/LConn1 -- RightUpper  Arm/RConn1
  Right Upper Arm COM/LConn1 -- RUACOM/RConn1
  Transform Sensor/RConn1 -- World Frame/RConn1
  Rotation Transform Right Arm/LConn1 -- Transform Sensor/RConn2

== system GolfSwing3D_SimscapePhysicalInterfaceSwitching/Right Wrist and Hand/RW Kinematically Driven ==
  RWConstraintTorqueLocal : nesl_utility/PS-Simulink Converter  PhysicalDomain=network_engine_domain  SubClassName=ps_output  LeftPortType=input  RightPortType=output  PseudoPeriodic=off  Frequencies=[]  VectorFormat=1-D array  Unit=inherit  AffineConversion=off
  RWForceLocal : nesl_utility/PS-Simulink Converter  PhysicalDomain=network_engine_domain  SubClassName=ps_output  LeftPortType=input  RightPortType=output  PseudoPeriodic=off  Frequencies=[]  VectorFormat=1-D array  Unit=inherit  AffineConversion=off
  RWTorqueLocal : nesl_utility/PS-Simulink Converter  PhysicalDomain=network_engine_domain  SubClassName=ps_output  LeftPortType=input  RightPortType=output  PseudoPeriodic=off  Frequencies=[]  VectorFormat=1-D array  Unit=inherit  AffineConversion=off
  RWTorqueXInput : nesl_utility/PS-Simulink Converter  PhysicalDomain=network_engine_domain  SubClassName=ps_output  LeftPortType=input  RightPortType=output  PseudoPeriodic=off  Frequencies=[]  VectorFormat=1-D array  Unit=inherit  AffineConversion=off
  RWTorqueYInput : nesl_utility/PS-Simulink Converter  PhysicalDomain=network_engine_domain  SubClassName=ps_output  LeftPortType=input  RightPortType=output  PseudoPeriodic=off  Frequencies=[]  VectorFormat=1-D array  Unit=inherit  AffineConversion=off
  "Right " : sm_lib/Joints/Universal Joint  JointMode=Normal  CompositeWrenchDir=BaseOnFollower  CompositeWrenchFrame=FollowerFrame  SenseConstraintForce=off  SenseConstraintTorque=on  SenseTotalForce=on  SenseTotalTorque=on  RxPositionTargetSpecify=off  RxPositionTargetPriority=Low  RxPositionTargetValue=RWStartPositionX  RxPositionTargetValueUnits=deg  RxVelocityTargetSpecify=off  RxVelocityTargetPriority=Low  RxVelocityTargetValue=RWStartVelocityX  RxVelocityTargetValueUnits=deg/s  RxEquilibriumPosition=0  RxEquilibriumPositionUnits=deg  RxSpringStiffness=0  RxSpringStiffnessUnits=N*m/deg  RxDampingCoefficient=0  RxDampingCoefficientUnits=N*m/(deg/s)  RxLowerLimitSpecify=off  RxLowerLimitBound=-90  RxLowerLimitBoundUnits=deg  RxLowerLimitStiffness=1e4  RxLowerLimitStiffnessUnits=N*m/deg  RxLowerLimitDamping=10  RxLowerLimitDampingUnits=N*m/(deg/s)  RxLowerLimitTransitionRegionWidth=0.1  RxLowerLimitTransitionRegionWidthUnits=deg  RxUpperLimitSpecify=off  RxUpperLimitBound=90  RxUpperLimitBoundUnits=deg  RxUpperLimitStiffness=1e4  RxUpperLimitStiffnessUnits=N*m/deg  RxUpperLimitDamping=10  RxUpperLimitDampingUnits=N*m/(deg/s)  RxUpperLimitTransitionRegionWidth=0.1  RxUpperLimitTransitionRegionWidthUnits=deg  RxTorqueActuationMode=ComputedTorque  RxMotionActuationMode=InputMotion  RxSensePosition=on  RxSenseVelocity=on  RxSenseAcceleration=off  RxSenseTorqueForce=on  RxSenseLowerLimitTorqueForce=off  RxSenseUpperLimitTorqueForce=off  RyPositionTargetSpecify=off  RyPositionTargetPriority=Low  RyPositionTargetValue=RWStartPositionY  RyPositionTargetValueUnits=deg  RyVelocityTargetSpecify=off  RyVelocityTargetPriority=Low  RyVelocityTargetValue=RWStartVelocityY  RyVelocityTargetValueUnits=deg/s  RyEquilibriumPosition=0  RyEquilibriumPositionUnits=deg  RySpringStiffness=0  RySpringStiffnessUnits=N*m/deg  RyDampingCoefficient=0  RyDampingCoefficientUnits=N*m/(deg/s)  RyLowerLimitSpecify=off  RyLowerLimitBound=-90  RyLowerLimitBoundUnits=deg  RyLowerLimitStiffness=1e4  RyLowerLimitStiffnessUnits=N*m/deg  RyLowerLimitDamping=10  RyLowerLimitDampingUnits=N*m/(deg/s)  RyLowerLimitTransitionRegionWidth=0.1  RyLowerLimitTransitionRegionWidthUnits=deg  RyUpperLimitSpecify=off  RyUpperLimitBound=90  RyUpperLimitBoundUnits=deg  RyUpperLimitStiffness=1e4  RyUpperLimitStiffnessUnits=N*m/deg  RyUpperLimitDamping=10  RyUpperLimitDampingUnits=N*m/(deg/s)  RyUpperLimitTransitionRegionWidth=0.1  RyUpperLimitTransitionRegionWidthUnits=deg  RyTorqueActuationMode=ComputedTorque  RyMotionActuationMode=InputMotion  RySensePosition=on  RySenseVelocity=on  RySenseAcceleration=off  RySenseTorqueForce=on  RySenseLowerLimitTorqueForce=off  RySenseUpperLimitTorqueForce=off
  RightWristPositionX : nesl_utility/PS-Simulink Converter  PhysicalDomain=network_engine_domain  SubClassName=ps_output  LeftPortType=input  RightPortType=output  PseudoPeriodic=off  Frequencies=[]  VectorFormat=1-D array  Unit=deg  AffineConversion=off
  RightWristPositionY : nesl_utility/PS-Simulink Converter  PhysicalDomain=network_engine_domain  SubClassName=ps_output  LeftPortType=input  RightPortType=output  PseudoPeriodic=off  Frequencies=[]  VectorFormat=1-D array  Unit=deg  AffineConversion=off
  RightWristVelocityX : nesl_utility/PS-Simulink Converter  PhysicalDomain=network_engine_domain  SubClassName=ps_output  LeftPortType=input  RightPortType=output  PseudoPeriodic=off  Frequencies=[]  VectorFormat=1-D array  Unit=deg/s  AffineConversion=off
  RightWristVelocityY : nesl_utility/PS-Simulink Converter  PhysicalDomain=network_engine_domain  SubClassName=ps_output  LeftPortType=input  RightPortType=output  PseudoPeriodic=off  Frequencies=[]  VectorFormat=1-D array  Unit=deg/s  AffineConversion=off
  Simulink-PS Converter25 : nesl_utility/Simulink-PS Converter  PhysicalDomain=network_engine_domain  SubClassName=ps_input  LeftPortType=input  RightPortType=output  PseudoPeriodic=off  Frequencies=[]  NoiseDistribution=none  NoiseParameters=[]  Unit=deg  AffineConversion=off  FilteringAndDerivatives=provide  SimscapeFilterOrder=1  InputFilterTimeConstant=0.001  UdotUserProvided=2
  Simulink-PS Converter27 : nesl_utility/Simulink-PS Converter  PhysicalDomain=network_engine_domain  SubClassName=ps_input  LeftPortType=input  RightPortType=output  PseudoPeriodic=off  Frequencies=[]  NoiseDistribution=none  NoiseParameters=[]  Unit=deg  AffineConversion=off  FilteringAndDerivatives=provide  SimscapeFilterOrder=1  InputFilterTimeConstant=0.001  UdotUserProvided=2
  Conn1 : PMIOPort  Side=Left
  RHGripStandoff : PMIOPort  Port=2  Side=Right
  tag scope: RWForceLocal=global, RWPositionX=global, RWPositionY=global, RWTorqueLocal=global, RWVelocityX=global, RWVelocityY=global
  wires:
  [FcnOutRWVelocityY] -> Simulink-PS Converter27/2
  [FcnOutRWPositionX] -> Simulink-PS Converter25/1
  [FcnOutRWAccelerationX] -> Simulink-PS Converter25/3
  [FcnOutRWPositionY] -> Simulink-PS Converter27/1
  [FcnOutRWVelocityX] -> Simulink-PS Converter25/2
  [FcnOutRWAccelerationY] -> Simulink-PS Converter27/3
  RightWristPositionY/1 -> [RWPositionY]  "RWPositionY"
  RightWristPositionX/1 -> [RWPositionX]  "RWPositionX"
  RightWristVelocityY/1 -> [RWVelocityY]  "RWVelocityY"
  RightWristVelocityX/1 -> [RWVelocityX]  "RWVelocityX"
  RWForceLocal/1 -> [RWForceLocal]  "RWForceLocal"
  RWTorqueLocal/1 -> [RWTorqueLocal]  "RWTorqueLocal"
  RWConstraintTorqueLocal/1 -> ?  "RWConstraintTorqueLocal"
  RWTorqueXInput/1 -> ?  "RWTorqueXInput"
  RWTorqueYInput/1 -> ?  "RWTorqueYInput"
  connections:
  "Right "/LConn2 -- Simulink-PS Converter25/RConn1
  "Right "/LConn1 -- Conn1/RConn1
  "Right "/LConn3 -- Simulink-PS Converter27/RConn1
  "Right "/RConn1 -- RHGripStandoff/RConn1
  RightWristPositionY/LConn1 -- "Right "/RConn5
  RWTorqueLocal/LConn1 -- "Right "/RConn10
  RightWristPositionX/LConn1 -- "Right "/RConn2
  RightWristVelocityY/LConn1 -- "Right "/RConn6
  RightWristVelocityX/LConn1 -- "Right "/RConn3
  RWForceLocal/LConn1 -- "Right "/RConn8
  RWConstraintTorqueLocal/LConn1 -- "Right "/RConn9
  RWTorqueXInput/LConn1 -- "Right "/RConn4
  RWTorqueYInput/LConn1 -- "Right "/RConn7
